simulink library "STPA_Library"  (Simulink 8.7)
settings: Solver=VariableStepAuto  SolverMode=SingleTasking  StartTime=0.0  StopTime=10.0  RelTol=1e-3

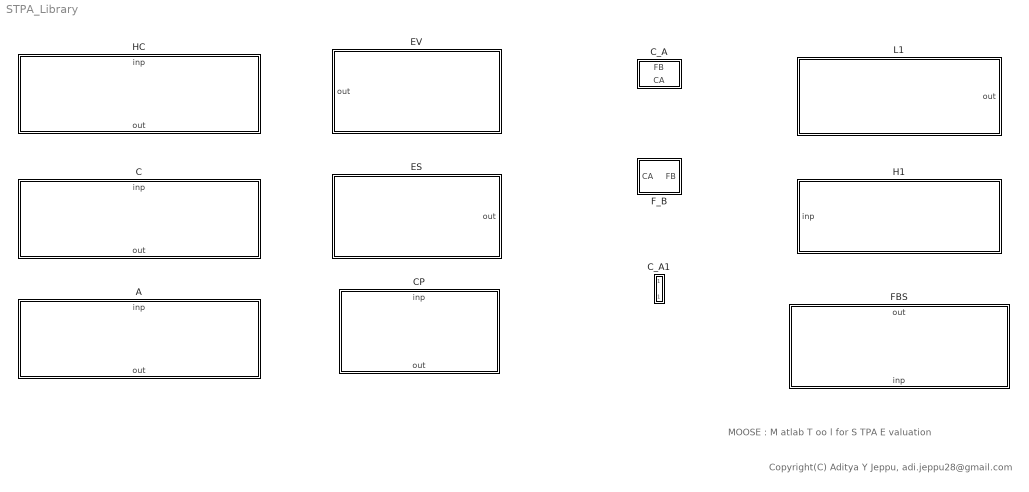
== system STPA_Library ==
  note: MOOSE : M atlab T oo l for S TPA E valuation
  note: Copyright(C) Aditya Y Jeppu, adi.jeppu28@gmail.com
  " FBS" : Subsystem  TreatAsAtomicUnit=on  mask(feedback_system){NAMEFORBLOCK=Wheel Brake Sensor, DES=Measure the outside \n air pressure and temperature}
      mask prompts: NAMEFORBLOCK "Provide a name"; DES "Provide a description of feedback system"
      mask help: Say what this feedback system does
      mask init:
      | set_param(gcb,'LinkStatus', 'none');
      settings: RTWFcnNameOpts=Use subsystem name  RTWFileNameOpts=Use function name
      mask DialogControl Control2 Prompt: ADD Input
      mask DialogControl Control2 Callback:
      | h = add_block('simulink/Sources/In1', [gcb '/inp'], 'MakeNameUnique', 'on');
      | hg = add_block('simulink/Sinks/Terminator', [gcb '/term'], 'MakeNameUnique', 'on');
      | hname = get_param(h,'PortHandles');
      | hgname = get_param(hg,'PortHandles');
      | add_line(gcb, hname.Outport(1), hgname.Inport(1));
      mask DialogControl Control3 Prompt: ADD Output
      mask DialogControl Control3 Callback:
      | h = add_block('simulink/Sinks/Out1', [gcb '/out'], 'MakeNameUnique', 'on');
      | hg = add_block('simulink/Sources/Ground', [gcb '/gnd'], 'MakeNameUnique', 'on');
      | hname = get_param(h,'PortHandles');
      | hgname = get_param(hg,'PortHandles');
      | add_line(gcb, hgname.Outport(1), hname.Inport(1));
      mask DialogControl Control4 Prompt: REM Input
      mask DialogControl Control4 Callback:
      | a=find_system(gcb,'SearchDepth',2,'LookUnderMasks','all','BlockType','Inport');
      | if ~isempty(a)
      | b=get_param(a{1},'PortConnectivity');
      | delete_block(a{1});
      | delete_block(b.DstBlock);
      | delete_line(find_system(gcb, 'SearchDepth',2,'LookUnderMasks','all','FindAll', 'on', 'Type', 'line', 'Connected', 'off'))
      | end
      mask DialogControl Control5 Prompt: REM Output
      mask DialogControl Control5 Callback:
      | a=find_system(gcb,'SearchDepth',2,'LookUnderMasks','all','BlockType','Outport');
      | if ~isempty(a)
      | b=get_param(a{1},'PortConnectivity');
      | delete_block(a{1});
      | delete_block(b.SrcBlock);
      | delete_line(find_system(gcb, 'SearchDepth',2,'LookUnderMasks','all','FindAll', 'on', 'Type', 'line', 'Connected', 'off'))
      | end
      mask Display: disp(['Feedback System \n' NAMEFORBLOCK ':\n' DES])
  A : Subsystem  TreatAsAtomicUnit=on  mask(actuator){NAMEFORBLOCK=Valves, DES=Opens the valve}
      mask prompts: NAMEFORBLOCK "Provide a name for Block"; DES "Provide a description of Responsibility"
      mask help: Say what this actuator does
      mask init:
      | set_param(gcb,'LinkStatus', 'none');
      settings: RTWFcnNameOpts=Use subsystem name  RTWFileNameOpts=Use function name
      mask DialogControl Control2 Prompt: ADD Input
      mask DialogControl Control2 Callback:
      | h = add_block('simulink/Sources/In1', [gcb '/inp'], 'MakeNameUnique', 'on');
      | hg = add_block('simulink/Sinks/Terminator', [gcb '/term'], 'MakeNameUnique', 'on');
      | hname = get_param(h,'PortHandles');
      | hgname = get_param(hg,'PortHandles');
      | add_line(gcb, hname.Outport(1), hgname.Inport(1));
      mask DialogControl Control3 Prompt: ADD Output
      mask DialogControl Control3 Callback:
      | h = add_block('simulink/Sinks/Out1', [gcb '/out'], 'MakeNameUnique', 'on');
      | hg = add_block('simulink/Sources/Ground', [gcb '/gnd'], 'MakeNameUnique', 'on');
      | hname = get_param(h,'PortHandles');
      | hgname = get_param(hg,'PortHandles');
      | add_line(gcb, hgname.Outport(1), hname.Inport(1));
      mask DialogControl Control4 Prompt: REM Input
      mask DialogControl Control4 Callback:
      | a=find_system(gcb,'SearchDepth',2,'LookUnderMasks','all','BlockType','Inport');
      | if ~isempty(a)
      | b=get_param(a{1},'PortConnectivity');
      | delete_block(a{1});
      | delete_block(b.DstBlock);
      | delete_line(find_system(gcb, 'SearchDepth',2,'LookUnderMasks','all','FindAll', 'on', 'Type', 'line', 'Connected', 'off'))
      | end
      mask DialogControl Control5 Prompt: REM Output
      mask DialogControl Control5 Callback:
      | a=find_system(gcb,'SearchDepth',2,'LookUnderMasks','all','BlockType','Outport');
      | if ~isempty(a)
      | b=get_param(a{1},'PortConnectivity');
      | delete_block(a{1});
      | delete_block(b.SrcBlock);
      | delete_line(find_system(gcb, 'SearchDepth',2,'LookUnderMasks','all','FindAll', 'on', 'Type', 'line', 'Connected', 'off'))
      | end
      mask Display: disp(['Actuator \n' NAMEFORBLOCK ':\n' DES])
  C : Subsystem  TreatAsAtomicUnit=on  mask(controller){NAMEFORBLOCK=The ABS Controller, DES=The controller controls the \n actuators}
      mask prompts: NAMEFORBLOCK "Provide a name for Block"; DES "Provide a description of Responsibility"
      mask help: Say what this controller does
      mask init:
      | set_param(gcb,'LinkStatus', 'none');
      settings: RTWFcnNameOpts=Use subsystem name  RTWFileNameOpts=Use function name
      mask DialogControl Control2 Prompt: ADD Input
      mask DialogControl Control2 Callback:
      | h = add_block('simulink/Sources/In1', [gcb '/inp'], 'MakeNameUnique', 'on');
      | hg = add_block('simulink/Sinks/Terminator', [gcb '/term'], 'MakeNameUnique', 'on');
      | hname = get_param(h,'PortHandles');
      | hgname = get_param(hg,'PortHandles');
      | add_line(gcb, hname.Outport(1), hgname.Inport(1));
      mask DialogControl Control3 Prompt: ADD Output
      mask DialogControl Control3 Callback:
      | h = add_block('simulink/Sinks/Out1', [gcb '/out'], 'MakeNameUnique', 'on');
      | hg = add_block('simulink/Sources/Ground', [gcb '/gnd'], 'MakeNameUnique', 'on');
      | hname = get_param(h,'PortHandles');
      | hgname = get_param(hg,'PortHandles');
      | add_line(gcb, hgname.Outport(1), hname.Inport(1));
      mask DialogControl Control4 Prompt: REM Input
      mask DialogControl Control4 Callback:
      | a=find_system(gcb,'SearchDepth',2,'LookUnderMasks','all','BlockType','Inport');
      | if ~isempty(a)
      | b=get_param(a{1},'PortConnectivity');
      | delete_block(a{1});
      | delete_block(b.DstBlock);
      | delete_line(find_system(gcb, 'SearchDepth',2,'LookUnderMasks','all','FindAll', 'on', 'Type', 'line', 'Connected', 'off'))
      | end
      mask DialogControl Control5 Prompt: REM Output
      mask DialogControl Control5 Callback:
      | a=find_system(gcb,'SearchDepth',2,'LookUnderMasks','all','BlockType','Outport');
      | if ~isempty(a)
      | b=get_param(a{1},'PortConnectivity');
      | delete_block(a{1});
      | delete_block(b.SrcBlock);
      | delete_line(find_system(gcb, 'SearchDepth',2,'LookUnderMasks','all','FindAll', 'on', 'Type', 'line', 'Connected', 'off'))
      | end
      mask Display: disp(['Controller \n' NAMEFORBLOCK ':\n' DES])
  CP : Subsystem  TreatAsAtomicUnit=on  mask(controlled_process){NAMEFORBLOCK=Automated Braking System, DES=Ensures smooth braking \n of vehicle}
      mask prompts: NAMEFORBLOCK "Provide a name for Block"; DES "Provide a description of Responsibility"
      mask help: Say what this controlled process does
      settings: RTWFcnNameOpts=Use subsystem name  RTWFileNameOpts=Use function name
      mask DialogControl Control2 Prompt: ADD Input
      mask DialogControl Control2 Callback:
      | set_param(gcb,'LinkStatus', 'none');
      | h = add_block('simulink/Sources/In1', [gcb '/inp'], 'MakeNameUnique', 'on');
      | hg = add_block('simulink/Sinks/Terminator', [gcb '/term'], 'MakeNameUnique', 'on');
      | hname = get_param(h,'PortHandles');
      | hgname = get_param(hg,'PortHandles');
      | add_line(gcb, hname.Outport(1), hgname.Inport(1));
      mask DialogControl Control3 Prompt: ADD Output
      mask DialogControl Control3 Callback:
      | set_param(gcb,'LinkStatus', 'none');
      | h = add_block('simulink/Sinks/Out1', [gcb '/out'], 'MakeNameUnique', 'on');
      | hg = add_block('simulink/Sources/Ground', [gcb '/gnd'], 'MakeNameUnique', 'on');
      | hname = get_param(h,'PortHandles');
      | hgname = get_param(hg,'PortHandles');
      | add_line(gcb, hgname.Outport(1), hname.Inport(1));
      mask DialogControl Control4 Prompt: REM Input
      mask DialogControl Control4 Callback:
      | set_param(gcb,'LinkStatus', 'none');
      | a=find_system(gcb,'SearchDepth',2,'LookUnderMasks','all','BlockType','Inport');
      | if ~isempty(a)
      | b=get_param(a{1},'PortConnectivity');
      | delete_block(a{1});
      | delete_block(b.DstBlock);
      | delete_line(find_system(gcb, 'SearchDepth',2,'LookUnderMasks','all','FindAll', 'on', 'Type', 'line', 'Connected', 'off'))
      | end
      mask DialogControl Control5 Prompt: REM Output
      mask DialogControl Control5 Callback:
      | set_param(gcb,'LinkStatus', 'none');
      | a=find_system(gcb,'SearchDepth',2,'LookUnderMasks','all','BlockType','Outport');
      | if ~isempty(a)
      | b=get_param(a{1},'PortConnectivity');
      | delete_block(a{1});
      | delete_block(b.SrcBlock);
      | delete_line(find_system(gcb, 'SearchDepth',2,'LookUnderMasks','all','FindAll', 'on', 'Type', 'line', 'Connected', 'off'))
      | end
      mask Display: disp(['Controlled Process \n' NAMEFORBLOCK ':\n' DES])
  C_A : Subsystem  TreatAsAtomicUnit=on  mask(control_action){DES=Sets the modes \n for the controller, UCA1=[#H1], UCA2=[#H1], UCA3=[#H1], UCA4=[#H1]}
      mask prompts: DES "Provide a description of Control Action"; UCA1 "Not providing causes hazard [link Hazard]"; UCA2 "Providing causes hazard [link Hazard]"; UCA3 "Too early, too late, out of order [link Hazard]"; UCA4 "Stopped too soon, applied too long [link Hazard]"
      mask help:
      | <Source> <Type> <Control Action> <Context> <Link to Hazards>
      | Source = System Above, Type = {provided, not provided ..], Control Action = command
      | from the description, Context = While/When .. Always link to a hazard
      mask init:
      | set_param(gcb,'LinkStatus', 'none');
      settings: AttributesFormatString=%<DES>  RTWFcnNameOpts=Use subsystem name  RTWFileNameOpts=Use function name
      mask Display: disp('ca')
  C_A1 : Subsystem  TreatAsAtomicUnit=on  mask(color_changer){}
      mask help: This just changes color to black
      mask init:
      | set_param(gcb,'LinkStatus', 'none');
      settings: RTWFcnNameOpts=Use subsystem name  RTWFileNameOpts=Use function name
      mask Display: disp(' ')
  ES : Subsystem  TreatAsAtomicUnit=on  mask(external_system){NAMEFORBLOCK=Accelerator, DES=The change in speed \n will effect braking}
      mask prompts: NAMEFORBLOCK "Provide a name for Block"; DES "Provide a description of the Interaction"
      mask help: Say how this external system interacts with the process
      mask init:
      | set_param(gcb,'LinkStatus', 'none');
      settings: RTWFcnNameOpts=Use subsystem name  RTWFileNameOpts=Use function name
      mask DialogControl Control2 Prompt: ADD Input
      mask DialogControl Control2 Callback:
      | h = add_block('simulink/Sources/In1', [gcb '/inp'], 'MakeNameUnique', 'on');
      | hg = add_block('simulink/Sinks/Terminator', [gcb '/term'], 'MakeNameUnique', 'on');
      | hname = get_param(h,'PortHandles');
      | hgname = get_param(hg,'PortHandles');
      | add_line(gcb, hname.Outport(1), hgname.Inport(1));
      mask DialogControl Control3 Prompt: ADD Output
      mask DialogControl Control3 Callback:
      | h = add_block('simulink/Sinks/Out1', [gcb '/out'], 'MakeNameUnique', 'on');
      | hg = add_block('simulink/Sources/Ground', [gcb '/gnd'], 'MakeNameUnique', 'on');
      | hname = get_param(h,'PortHandles');
      | hgname = get_param(hg,'PortHandles');
      | add_line(gcb, hgname.Outport(1), hname.Inport(1));
      mask DialogControl Control4 Prompt: REM Input
      mask DialogControl Control4 Callback:
      | a=find_system(gcb,'SearchDepth',2,'LookUnderMasks','all','BlockType','Inport');
      | if ~isempty(a)
      | b=get_param(a{1},'PortConnectivity');
      | delete_block(a{1});
      | delete_block(b.DstBlock);
      | delete_line(find_system(gcb, 'SearchDepth',2,'LookUnderMasks','all','FindAll', 'on', 'Type', 'line', 'Connected', 'off'))
      | end
      mask DialogControl Control5 Prompt: REM Output
      mask DialogControl Control5 Callback:
      | a=find_system(gcb,'SearchDepth',2,'LookUnderMasks','all','BlockType','Outport');
      | if ~isempty(a)
      | b=get_param(a{1},'PortConnectivity');
      | delete_block(a{1});
      | delete_block(b.SrcBlock);
      | delete_line(find_system(gcb, 'SearchDepth',2,'LookUnderMasks','all','FindAll', 'on', 'Type', 'line', 'Connected', 'off'))
      | end
      mask Display: disp(['External System \n' NAMEFORBLOCK ':\n' DES])
  EV : Subsystem  TreatAsAtomicUnit=on  mask(environment){NAMEFORBLOCK=Road, DES=The road friction \n effects the braking}
      mask prompts: NAMEFORBLOCK "Provide a name for Block"; DES "Provide a description of Interaction"
      mask help: Say how this environment interacts with the system
      mask init:
      | set_param(gcb,'LinkStatus', 'none');
      settings: RTWFcnNameOpts=Use subsystem name  RTWFileNameOpts=Use function name
      mask DialogControl Control2 Prompt: ADD Input
      mask DialogControl Control2 Callback:
      | h = add_block('simulink/Sources/In1', [gcb '/inp'], 'MakeNameUnique', 'on');
      | hg = add_block('simulink/Sinks/Terminator', [gcb '/term'], 'MakeNameUnique', 'on');
      | hname = get_param(h,'PortHandles');
      | hgname = get_param(hg,'PortHandles');
      | add_line(gcb, hname.Outport(1), hgname.Inport(1));
      mask DialogControl Control3 Prompt: ADD Output
      mask DialogControl Control3 Callback:
      | h = add_block('simulink/Sinks/Out1', [gcb '/out'], 'MakeNameUnique', 'on');
      | hg = add_block('simulink/Sources/Ground', [gcb '/gnd'], 'MakeNameUnique', 'on');
      | hname = get_param(h,'PortHandles');
      | hgname = get_param(hg,'PortHandles');
      | add_line(gcb, hgname.Outport(1), hname.Inport(1));
      mask DialogControl Control4 Prompt: REM Input
      mask DialogControl Control4 Callback:
      | a=find_system(gcb,'SearchDepth',2,'LookUnderMasks','all','BlockType','Inport');
      | if ~isempty(a)
      | b=get_param(a{1},'PortConnectivity');
      | delete_block(a{1});
      | delete_block(b.DstBlock);
      | delete_line(find_system(gcb, 'SearchDepth',2,'LookUnderMasks','all','FindAll', 'on', 'Type', 'line', 'Connected', 'off'))
      | end
      mask DialogControl Control5 Prompt: REM Output
      mask DialogControl Control5 Callback:
      | a=find_system(gcb,'SearchDepth',2,'LookUnderMasks','all','BlockType','Outport');
      | if ~isempty(a)
      | b=get_param(a{1},'PortConnectivity');
      | delete_block(a{1});
      | delete_block(b.SrcBlock);
      | delete_line(find_system(gcb, 'SearchDepth',2,'LookUnderMasks','all','FindAll', 'on', 'Type', 'line', 'Connected', 'off'))
      | end
      mask Display: disp(['Environment \n' NAMEFORBLOCK ':\n' DES])
  F_B : Subsystem  TreatAsAtomicUnit=on  mask(feedback){DES=Wheel \n speed}
      mask prompts: DES "Provide a description"
      mask help: Say what this feeds back from the system
      mask init:
      | set_param(gcb,'LinkStatus', 'none');
      settings: AttributesFormatString=%<DES>  RTWFcnNameOpts=Use subsystem name  RTWFileNameOpts=Use function name
      mask Display: disp('fb')
  H1 : Subsystem  TreatAsAtomicUnit=on  mask(hazard){NAMEFORBLOCK=Hazard 01, DES=Inadvertent movement of vehicle}
      mask prompts: NAMEFORBLOCK "Provide a name for Block"; DES "Provide a description of Hazard"
      mask help: Provide details of the Hazard
      mask init:
      | set_param(gcb,'LinkStatus', 'none');
      settings: RTWFcnNameOpts=Use subsystem name  RTWFileNameOpts=Use function name
      mask DialogControl Control2 Prompt: ADD Input
      mask DialogControl Control2 Callback:
      | h = add_block('simulink/Sources/In1', [gcb '/inp'], 'MakeNameUnique', 'on');
      | hg = add_block('simulink/Sinks/Terminator', [gcb '/term'], 'MakeNameUnique', 'on');
      | hname = get_param(h,'PortHandles');
      | hgname = get_param(hg,'PortHandles');
      | add_line(gcb, hname.Outport(1), hgname.Inport(1));
      mask DialogControl Control3 Prompt: ADD Output
      mask DialogControl Control3 Callback:
      | h = add_block('simulink/Sinks/Out1', [gcb '/out'], 'MakeNameUnique', 'on');
      | hg = add_block('simulink/Sources/Ground', [gcb '/gnd'], 'MakeNameUnique', 'on');
      | hname = get_param(h,'PortHandles');
      | hgname = get_param(hg,'PortHandles');
      | add_line(gcb, hgname.Outport(1), hname.Inport(1));
      mask DialogControl Control4 Prompt: REM Input
      mask DialogControl Control4 Callback:
      | a=find_system(gcb,'SearchDepth',2,'LookUnderMasks','all','BlockType','Inport');
      | if ~isempty(a)
      | b=get_param(a{1},'PortConnectivity');
      | delete_block(a{1});
      | delete_block(b.DstBlock);
      | delete_line(find_system(gcb, 'SearchDepth',2,'LookUnderMasks','all','FindAll', 'on', 'Type', 'line', 'Connected', 'off'))
      | end
      mask DialogControl Control5 Prompt: REM Output
      mask DialogControl Control5 Callback:
      | a=find_system(gcb,'SearchDepth',2,'LookUnderMasks','all','BlockType','Outport');
      | if ~isempty(a)
      | b=get_param(a{1},'PortConnectivity');
      | delete_block(a{1});
      | delete_block(b.SrcBlock);
      | delete_line(find_system(gcb, 'SearchDepth',2,'LookUnderMasks','all','FindAll', 'on', 'Type', 'line', 'Connected', 'off'))
      | end
      mask Display: disp(['Hazard \n' NAMEFORBLOCK ':\n' DES])
  HC : Subsystem  TreatAsAtomicUnit=on  mask(human_controller){NAMEFORBLOCK=Driver, DES=The Driver controls the \n ABS system}
      mask prompts: NAMEFORBLOCK "Provide a name for Block"; DES "Provide a description of Responsibility"
      mask help: Say what this human controller does
      mask init:
      | set_param(gcb,'LinkStatus','none')
      settings: RTWFcnNameOpts=Use subsystem name  RTWFileNameOpts=Use function name
      mask DialogControl Control2 Prompt: ADD Input
      mask DialogControl Control2 Callback:
      | h = add_block('simulink/Sources/In1', [gcb '/inp'], 'MakeNameUnique', 'on');
      | hg = add_block('simulink/Sinks/Terminator', [gcb '/term'], 'MakeNameUnique', 'on');
      | hname = get_param(h,'PortHandles');
      | hgname = get_param(hg,'PortHandles');
      | add_line(gcb, hname.Outport(1), hgname.Inport(1));
      mask DialogControl Control3 Prompt: ADD Output
      mask DialogControl Control3 Callback:
      | h = add_block('simulink/Sinks/Out1', [gcb '/out'], 'MakeNameUnique', 'on');
      | hg = add_block('simulink/Sources/Ground', [gcb '/gnd'], 'MakeNameUnique', 'on');
      | hname = get_param(h,'PortHandles');
      | hgname = get_param(hg,'PortHandles');
      | add_line(gcb, hgname.Outport(1), hname.Inport(1));
      mask DialogControl Control4 Prompt: REM Input
      mask DialogControl Control4 Callback:
      | a=find_system(gcb,'SearchDepth',2,'LookUnderMasks','all','BlockType','Inport');
      | if ~isempty(a)
      | b=get_param(a{1},'PortConnectivity');
      | delete_block(a{1});
      | delete_block(b.DstBlock);
      | delete_line(find_system(gcb, 'SearchDepth',2,'LookUnderMasks','all','FindAll', 'on', 'Type', 'line', 'Connected', 'off'))
      | end
      mask DialogControl Control5 Prompt: REM Output
      mask DialogControl Control5 Callback:
      | a=find_system(gcb,'SearchDepth',2,'LookUnderMasks','all','BlockType','Outport');
      | if ~isempty(a)
      | b=get_param(a{1},'PortConnectivity');
      | delete_block(a{1});
      | delete_block(b.SrcBlock);
      | delete_line(find_system(gcb, 'SearchDepth',2,'LookUnderMasks','all','FindAll', 'on', 'Type', 'line', 'Connected', 'off'))
      | end
      mask Display: disp(['Human Controller \n' NAMEFORBLOCK ':\n' DES])
  L1 : Subsystem  TreatAsAtomicUnit=on  mask(loss){NAMEFORBLOCK=Loss 01, DES=The cabin ruptures – structural \n damage causing loss of life/injury \n– even death, LOSSCAT=1}
      mask prompts: NAMEFORBLOCK "Provide a name for Block"; DES "Provide a description of Loss"; LOSSCAT "Provide Loss Category CAT 1, 2, 3"
      mask help: Provide details of the loss
      mask init:
      | set_param(gcb,'LinkStatus', 'none');
      settings: AttributesFormatString=CAT %<LOSSCAT>  RTWFcnNameOpts=Use subsystem name  RTWFileNameOpts=Use function name
      mask DialogControl Control3 Prompt: ADD Output
      mask DialogControl Control3 Callback:
      | h = add_block('simulink/Sinks/Out1', [gcb '/out'], 'MakeNameUnique', 'on');
      | hg = add_block('simulink/Sources/Ground', [gcb '/gnd'], 'MakeNameUnique', 'on');
      | hname = get_param(h,'PortHandles');
      | hgname = get_param(hg,'PortHandles');
      | add_line(gcb, hgname.Outport(1), hname.Inport(1));
      mask DialogControl Control5 Prompt: REM Output
      mask DialogControl Control5 Callback:
      | a=find_system(gcb,'SearchDepth',2,'LookUnderMasks','all','BlockType','Outport');
      | if ~isempty(a)
      | b=get_param(a{1},'PortConnectivity');
      | delete_block(a{1});
      | delete_block(b.SrcBlock);
      | delete_line(find_system(gcb, 'SearchDepth',2,'LookUnderMasks','all','FindAll', 'on', 'Type', 'line', 'Connected', 'off'))
      | end
      mask Display: disp(['Loss \n' NAMEFORBLOCK ':\n' DES])

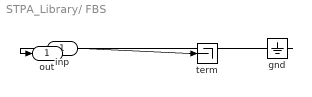
== system STPA_Library/ FBS ==
  inp : Inport
  gnd : Ground
  term : Terminator
  out : Outport
  wires:
  inp/1 -> term/1
  gnd/1 -> out/1

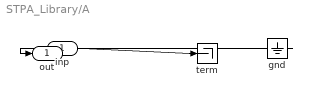
== system STPA_Library/A ==
  inp : Inport
  gnd : Ground
  term : Terminator
  out : Outport
  wires:
  gnd/1 -> out/1
  inp/1 -> term/1

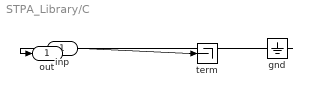
== system STPA_Library/C ==
  inp : Inport
  gnd : Ground
  term : Terminator
  out : Outport
  wires:
  inp/1 -> term/1
  gnd/1 -> out/1

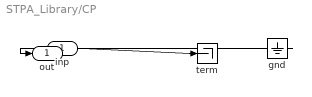
== system STPA_Library/CP ==
  inp : Inport
  gnd : Ground
  term : Terminator
  out : Outport
  wires:
  gnd/1 -> out/1
  inp/1 -> term/1

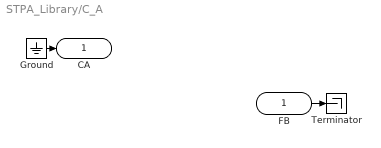
== system STPA_Library/C_A ==
  FB : Inport
      mask Display:
      | plot([0 60-10],[0 0]);
      | plot([0 0],[0 16]);
      | plot([0 60-10],[16 16]);
      | plot([60-10 60],[16 8]);
      | plot([60-10 60],[0 8]);
  Ground : Ground
  Terminator : Terminator
  CA : Outport
      mask Display:
      | plot([10 65],[0 0]);
      | plot([65-1 65-1],[0 16]);
      | plot([10 65],[16 16]);
      | plot([0 10],[8 16]);
      | plot([0 10],[8 0]);
  wires:
  Ground/1 -> CA/1
  FB/1 -> Terminator/1

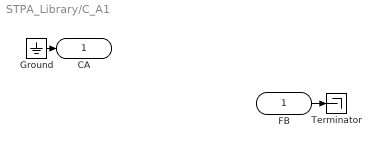
== system STPA_Library/C_A1 ==
  FB : Inport
      mask Display:
      | plot([0 60-10],[0 0]);
      | plot([0 0],[0 16]);
      | plot([0 60-10],[16 16]);
      | plot([60-10 60],[16 8]);
      | plot([60-10 60],[0 8]);
  Ground : Ground
  Terminator : Terminator
  CA : Outport
      mask Display:
      | plot([10 65],[0 0]);
      | plot([65-1 65-1],[0 16]);
      | plot([10 65],[16 16]);
      | plot([0 10],[8 16]);
      | plot([0 10],[8 0]);
  wires:
  Ground/1 -> CA/1
  FB/1 -> Terminator/1

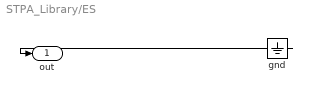
== system STPA_Library/ES ==
  gnd : Ground
  out : Outport
  wires:
  gnd/1 -> out/1

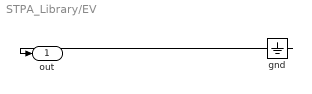
== system STPA_Library/EV ==
  gnd : Ground
  out : Outport
  wires:
  gnd/1 -> out/1

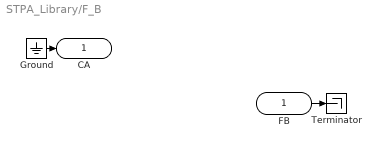
== system STPA_Library/F_B ==
  FB : Inport
      mask Display:
      | plot([0 60-10],[0 0]);
      | plot([0 0],[0 16]);
      | plot([0 60-10],[16 16]);
      | plot([60-10 60],[16 8]);
      | plot([60-10 60],[0 8]);
  Ground : Ground
  Terminator : Terminator
  CA : Outport
      mask Display:
      | plot([10 65],[0 0]);
      | plot([65-1 65-1],[0 16]);
      | plot([10 65],[16 16]);
      | plot([0 10],[8 16]);
      | plot([0 10],[8 0]);
  wires:
  FB/1 -> Terminator/1
  Ground/1 -> CA/1

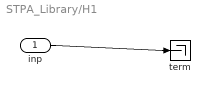
== system STPA_Library/H1 ==
  inp : Inport
  term : Terminator
  wires:
  inp/1 -> term/1

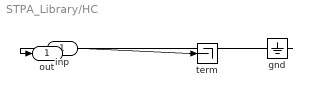
== system STPA_Library/HC ==
  inp : Inport
  gnd : Ground
  term : Terminator
  out : Outport
  wires:
  gnd/1 -> out/1
  inp/1 -> term/1

== system STPA_Library/L1 ==
  gnd : Ground
  out : Outport
  wires:
  gnd/1 -> out/1
